simulink model "ant_spring_const_l0"  (R2020b)
settings: Solver=ode4  StartTime=0.0  StopTime=40  FixedStep=0.001  RelTol=1e-3
model workspace (MAT data in the model file):
  l0 = [0.189353021319; 0.189353021319; 0.583222456778; 0.583222456778; 0.682071526229; 0.682071526229]
  p1_sol = [-196.46190846; -196.46190846; -196.46190846; -196.46190846; -196.46190846; 244.7265907; 244.7265907; 244.7265907; 244.7265907; 244.7265907; 0.108119886166; 0.108119886166; 0.108119886166; 0.108119886166; 0.108119886166]
  p2_sol = [-39.726939819; -163.425908656; -189.145615997; -193.604265592; -219.559697571; 44.5746374772; 153.533472233; 68.0096135047; 63.0706600389; 365.58131095; 0.927523422495; 0.37135489076; 0.295363504694; 0.295780130224; 0.415380975864]
  p3_sol = [-152.907364382; -153.38439627; -153.384182952; -153.387392656; -153.387514498; 82.883192474; 156.637043328; 156.637072219; 156.662654025; 156.665094103; 0.0711552458823; 0.16264087768; 0.162640870132; 0.162634189747; 0.16263355254]
settings Model: OrderedModelArguments=off  Creator=dennis  LastModifiedBy=dennis

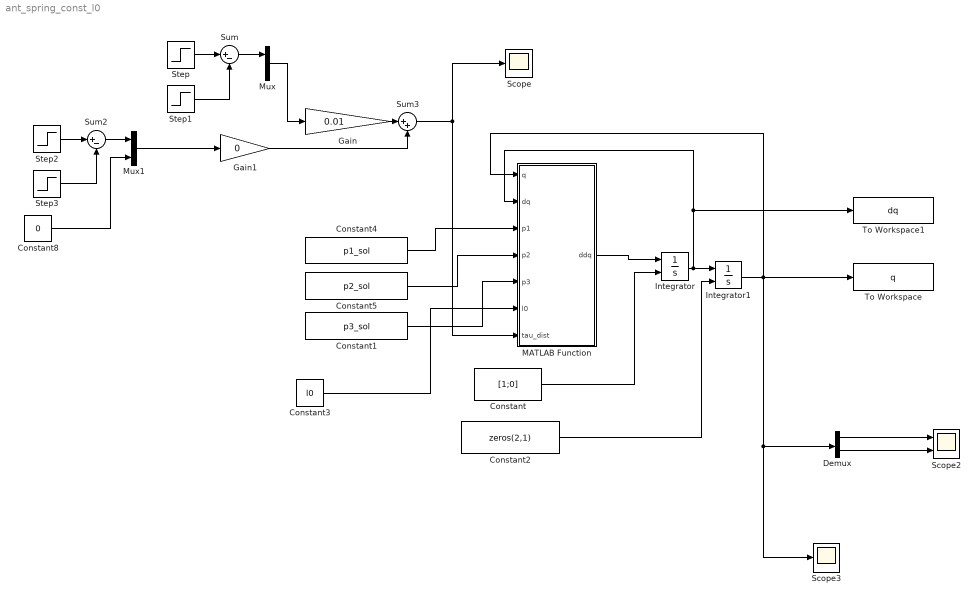
== system ant_spring_const_l0 ==
  Constant : Constant  Value=[1;0]
  Constant1 : Constant  Value=p3_sol
  Constant2 : Constant  Value=zeros(2,1)
  Constant3 : Constant  Value=l0
  Constant4 : Constant  Value=p1_sol
  Constant5 : Constant  Value=p2_sol
  Constant8 : Constant  Value=0
  Demux : Demux  Outputs=2
  Gain : Gain  Gain=0.01
  Gain1 : Gain  Gain=0
  Integrator : Integrator  InitialConditionSource=external
  Integrator1 : Integrator  InitialConditionSource=external
  MATLAB Function : MATLAB Function  TreatAsAtomicUnit=on
  Mux : Mux  Inputs=2
  Mux1 : Mux  Inputs=2
  Scope : Scope
  Scope2 : Scope  NumInputPorts=2
  Scope3 : Scope
  Step : Step  SampleTime=0
  Step1 : Step  Time=1.1  SampleTime=0
  Step2 : Step  Time=10  SampleTime=0
  Step3 : Step  Time=10.1  SampleTime=0
  Sum : Sum  Inputs=|+-
  Sum2 : Sum  Inputs=|+-
  Sum3 : Sum  Inputs=|++
  To Workspace : ToWorkspace  VariableName=q  SaveFormat=Timeseries  SampleTime=-1
  To Workspace1 : ToWorkspace  VariableName=dq  SaveFormat=Timeseries  SampleTime=-1
  wires:
  MATLAB Function/1(ddq) -> Integrator/1
  Integrator1/1 -> Scope3/1, Demux/1, MATLAB Function/1(q), To Workspace/1
  Demux/1 -> Scope2/1
  Demux/2 -> Scope2/2
  Constant5/1 -> MATLAB Function/4(p2)
  Constant2/1 -> Integrator1/2
  Integrator/1 -> To Workspace1/1, MATLAB Function/2(dq), Integrator1/1
  Constant/1 -> Integrator/2
  Mux/1 -> Gain/1
  Sum/1 -> Mux/1
  Step/1 -> Sum/1
  Step1/1 -> Sum/2
  Sum2/1 -> Mux1/1
  Step3/1 -> Sum2/2
  Step2/1 -> Sum2/1
  Gain/1 -> Sum3/1
  Sum3/1 -> MATLAB Function/7(tau_dist), Scope/1
  Mux1/1 -> Gain1/1
  Gain1/1 -> Sum3/2
  Constant8/1 -> Mux1/2
  Constant4/1 -> MATLAB Function/3(p1)
  Constant1/1 -> MATLAB Function/5(p3)
  Constant3/1 -> MATLAB Function/6(l0)

== matlab function ant_spring_const_l0/MATLAB Function ==
  data: q input; dq input; p1 input; ddq output; p2 input; p3 input; l0 input; tau_dist input
function ddq   = fcn(q,dq,p1,p2,p3,l0, tau_dist)


C = get_C(q,dq);
%G = get_G(q);
M = get_M(q);
%l0 = get_l(zeros(2,1));
n_w = 5;
l = get_l(q);
 Delta_l = l0 - l;


          F= [rbf_sym(Delta_l(1), p1(1:n_w),p1(n_w+1:2*n_w),p1(2*n_w+1:3*n_w));
        rbf_sym(Delta_l(2), p1(1:n_w),p1(n_w+1:2*n_w),p1(2*n_w+1:3*n_w));
        rbf_sym(Delta_l(3), p2(1:n_w),p2(n_w+1:2*n_w),p2(2*n_w+1:3*n_w));
        rbf_sym(Delta_l(4), p2(1:n_w),p2(n_w+1:2*n_w),p2(2*n_w+1:3*n_w));
        rbf_sym(Delta_l(5), p3(1:n_w),p3(n_w+1:2*n_w),p3(2*n_w+1:3*n_w));
        rbf_sym(Delta_l(6), p3(1:n_w),p3(n_w+1:2*n_w),p3(2*n_w+1:3*n_w))];
    
    tau = get_tau_F(q,F);

ddq = M\ (tau + tau_dist -C*dq);

end
